simulink model "IRB140_speed"  (R2019a)
settings: Solver=VariableStepAuto  StartTime=0.0  StopTime=10.0  RelTol=1e-3
InitFcn:
  | rpm_max=5000;
  | trq_stall=7;
  | T_i=1e-3;
  | eta=100;
  | rpm_eta=3000;
  | trq_eta=2.07;
  | J=0.672*1e-4;
  | rpm0=0;
  | gearRatio=10;
  | ts=0.0025;
undefined symbols (not defined in the file or in its folder): sigbuilder_block, X, Y, Z
libraries: sm_lib x61, fl_lib x37, nesl_utility x31, simulink x12, eeGeneralControl x12, ee_lib x6
(part 1 of 3)
settings Model: Creator=Richard urben  LastModifiedBy=Richard urben

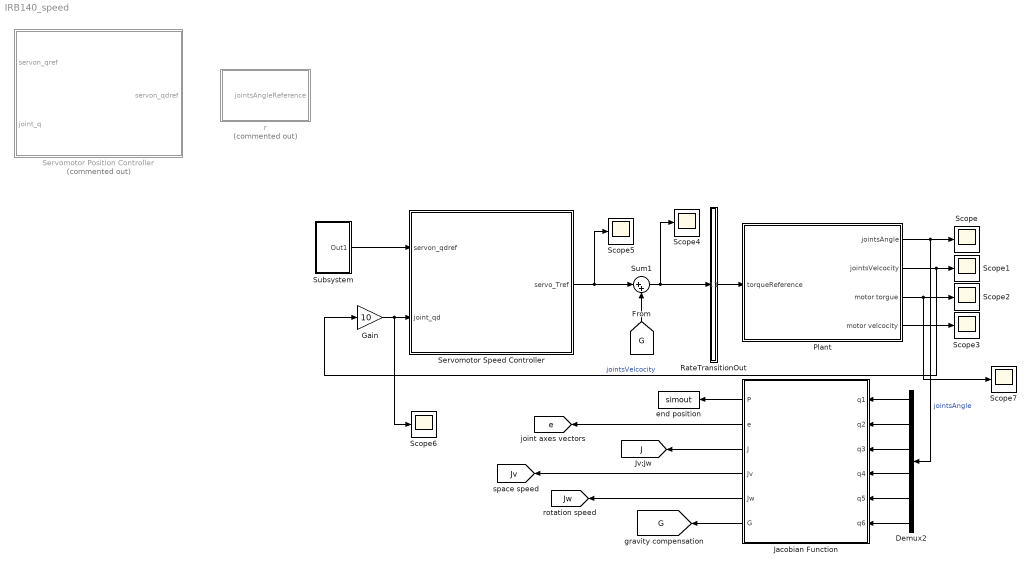
== system IRB140_speed ==
  Demux2 : Demux  Outputs=6
  Gain : Gain  Gain=10
  Jacobian Function : MATLAB Function  TreatAsAtomicUnit=on
  Plant : Subsystem
  RateTransitionOut : Subsystem
  Scope{,1..7} (8 alike) : Scope
  Servomotor Position Controller : Subsystem  Commented=on
  Servomotor Speed Controller : Subsystem
  Subsystem : Subsystem
  Sum1 : Sum  Inputs=|++
  "end position " : ToWorkspace  VariableName=simout  SaveFormat=Timeseries  SampleTime=-1
  r : Subsystem  Commented=on
      mask Display: disp('input')
  tag scope: G=global, J=global, Jv=global, Jw=global, e=global
  wires:
  Plant/2(jointsVelcocity) -> Gain/1, Scope1/1  "jointsVelcocity"
  RateTransitionOut/1(tRef) -> Plant/1(torqueReference)
  Plant/1(jointsAngle) -> Demux2/1, Scope/1  "jointsAngle"
  Plant/3(motor torgue) -> Scope7/1, Scope2/1
  Plant/4(motor velcocity) -> Scope3/1
  Demux2/5 -> Jacobian Function/5(q5)
  Demux2/3 -> Jacobian Function/3(q3)
  Demux2/2 -> Jacobian Function/2(q2)
  Demux2/4 -> Jacobian Function/4(q4)
  Demux2/1 -> Jacobian Function/1(q1)
  Demux2/6 -> Jacobian Function/6(q6)
  Jacobian Function/1(P) -> "end position "/1
  Jacobian Function/2(e) -> [e]
  Jacobian Function/3(J) -> [J]
  Jacobian Function/4(Jv) -> [Jv]
  Jacobian Function/5(Jw) -> [Jw]
  Jacobian Function/6(G) -> [G]
  Sum1/1 -> Scope4/1, RateTransitionOut/1(tRefIn)
  Servomotor Speed Controller/1(servo_Tref) -> Scope5/1, Sum1/1
  [G] -> Sum1/2
  Gain/1 -> Scope6/1, Servomotor Speed Controller/2(joint_qd)
  Subsystem/1(Out1) -> Servomotor Speed Controller/1(servon_qdref)

== system IRB140_speed/Plant ==
  torqueReference : Inport  Unit=N*m
  DC Voltage Source : fl_lib/Electrical/Electrical Sources/DC Voltage Source  v0=12 V
  ERef Vcc : fl_lib/Electrical/Electrical Elements/Electrical Reference
      settings: SourceProductName=Foundation Library
  MRRef Motor : fl_lib/Mechanical/Rotational Elements/Mechanical Rotational Reference
      settings: SourceProductName=Foundation Library
  robot : Subsystem
  servo system : Subsystem
  jointsAngle : Outport  Unit=deg
  jointsVelcocity : Outport  Port=2  Unit=deg/s
  motor torgue : Outport  Port=3
  motor velcocity : Outport  Port=4
  wires:
  robot/2(w) -> jointsVelcocity/1  "jointsvelocity"
  robot/1(q) -> jointsAngle/1  "jointsangle"
  servo system/1(torque) -> motor torgue/1  "motor torque"
  servo system/2(motVel) -> motor velcocity/1  "motor velocity"
  torqueReference/1 -> servo system/1(tRef)
  connections:
  robot/LConn4 -- servo system/RConn4
  robot/LConn5 -- servo system/RConn5
  robot/LConn3 -- servo system/RConn3
  robot/LConn1 -- servo system/RConn1
  robot/LConn6 -- servo system/RConn6
  servo system/RConn7 -- MRRef Motor/LConn1 -- robot/LConn7
  robot/LConn2 -- servo system/RConn2
  ERef Vcc/LConn1 -- DC Voltage Source/RConn1 -- servo system/LConn2
  DC Voltage Source/LConn1 -- servo system/LConn1

== system IRB140_speed/RateTransitionOut ==
  tRefIn : Inport  Unit=N*m
  Demux : Demux  Outputs=6
  Mux : Mux  Inputs=6
  Zero-Order Hold{,1..5} (6 alike) : ZeroOrderHold  SampleTime=-1
  tRef : Outport  SampleTime=0
  wires:
  Demux/3 -> Zero-Order Hold2/1
  tRefIn/1 -> Demux/1
  Demux/2 -> Zero-Order Hold1/1
  Demux/5 -> Zero-Order Hold4/1
  Demux/4 -> Zero-Order Hold3/1
  Demux/1 -> Zero-Order Hold/1
  Demux/6 -> Zero-Order Hold5/1
  Zero-Order Hold5/1 -> Mux/6
  Zero-Order Hold4/1 -> Mux/5
  Zero-Order Hold1/1 -> Mux/2
  Zero-Order Hold/1 -> Mux/1
  Zero-Order Hold2/1 -> Mux/3
  Zero-Order Hold3/1 -> Mux/4
  Mux/1 -> tRef/1

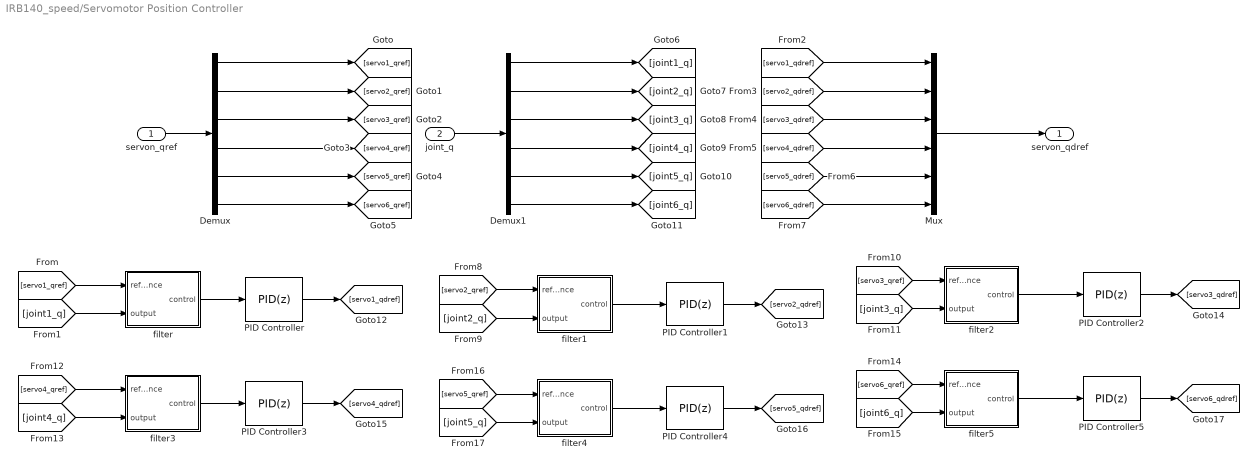
== system IRB140_speed/Servomotor Position Controller ==
  servon_qref : Inport  Unit=deg
  joint_q : Inport  Port=2  Unit=deg
  Demux : Demux  Outputs=6
  Demux1 : Demux  Outputs=6
  Mux : Mux  Inputs=6
  PID Controller : simulink/Continuous/PID Controller  Controller=PID  Form=Parallel  TimeDomain=Discrete-time  SampleTime=ts  IntegratorMethod=Forward Euler  FilterMethod=Forward Euler  ControllerParametersSource=internal  P=10.4951083286152  I=0.000420166597419455  D=-67.8994259865588  UseFilter=on  N=0.00133454786069086  TunerSelectOption=Transfer Function Based (PID Tuner App)  InitialConditionSource=internal  InitialConditionForIntegrator=0  InitialConditionForFilter=0  DifferentiatorICPrevScaledInput=0  ExternalReset=none  TrackingMode=off  Kt=1  LimitOutput=off  UpperSaturationLimit=inf  LowerSaturationLimit=-inf  LinearizeAsGain=on  AntiWindupMode=none  Kb=1  POutMin=[]  POutMax=[]  IOutMin=[]  IOutMax=[]  DOutMin=[]  DOutMax=[]  NOutMin=[]  NOutMax=[]  SumOutMin=[]  SumOutMax=[]  SaturationOutMin=[]  SaturationOutMax=[]  PParamMin=[]  PParamMax=[]  IParamMin=[]  IParamMax=[]  DParamMin=[]  DParamMax=[]  NParamMin=[]  NParamMax=[]  KbParamMin=[]  KbParamMax=[]  KtParamMin=[]  KtParamMax=[]  KbOutMin=[]  KbOutMax=[]  KtOutMin=[]  KtOutMax=[]  IntegratorOutMin=[]  IntegratorOutMax=[]  FilterOutMin=[]  FilterOutMax=[]  SumI1OutMin=[]  SumI1OutMax=[]  SumI2OutMin=[]  SumI2OutMax=[]  SumI3OutMin=[]  SumI3OutMax=[]  SumI4OutMin=[]  SumI4OutMax=[]  SumDOutMin=[]  SumDOutMax=[]  DifferentiatorOutMin=[]  DifferentiatorOutMax=[]  FilterDiffOutCoefMin=[]  FilterDiffOutCoefMax=[]  ReciprocalOutMin=[]  ReciprocalOutMax=[]  SumDenOutMin=[]  SumDenOutMax=[]  SumNumOutMin=[]  SumNumOutMax=[]  DivideOutMin=[]  DivideOutMax=[]  IntegratorContinuousStateAttributes=''  IntegratorStateMustResolveToSignalObject=off  IntegratorRTWStateStorageClass=Auto  FilterContinuousStateAttributes=''  FilterStateMustResolveToSignalObject=off  FilterRTWStateStorageClass=Auto  ParallelPVariant=InternalParameters  IdealPVariant=Disabled  IVariant=InternalParameters  DVariant=InternalParameters  IntegratorVariant=Discrete  SatVariant=Disabled  AWVariant=Passthrough  PCopyVariant=Disabled  TRVariant=Disabled  FdbkBlocksVariant=Forward  IdealPFdbkVariant=Disabled  SatFdbkVariant=Disabled  DerivativeFilterVariant=ForwardEulerFilter  NVariant=InternalParameters  NCopyVariant=Disabled  FilterICVariant=InternalICsFilter  IntegratorICVariant=InternalICs  ExternalResetVariant=Disabled  TRSumVariant=Passthrough  SumFdbkVariant=Disabled  SumVariant=Sum_PID
  PID Controller1 : simulink/Continuous/PID Controller  Controller=PID  Form=Parallel  TimeDomain=Discrete-time  SampleTime=ts  IntegratorMethod=Forward Euler  FilterMethod=Forward Euler  ControllerParametersSource=internal  P=3.54979973257463  I=0.000142016761735363  D=5.15669282783303  UseFilter=on  N=761.904761904762  TunerSelectOption=Transfer Function Based (PID Tuner App)  InitialConditionSource=internal  InitialConditionForIntegrator=0  InitialConditionForFilter=0  DifferentiatorICPrevScaledInput=0  ExternalReset=none  TrackingMode=off  Kt=1  LimitOutput=off  UpperSaturationLimit=inf  LowerSaturationLimit=-inf  LinearizeAsGain=on  AntiWindupMode=none  Kb=1  POutMin=[]  POutMax=[]  IOutMin=[]  IOutMax=[]  DOutMin=[]  DOutMax=[]  NOutMin=[]  NOutMax=[]  SumOutMin=[]  SumOutMax=[]  SaturationOutMin=[]  SaturationOutMax=[]  PParamMin=[]  PParamMax=[]  IParamMin=[]  IParamMax=[]  DParamMin=[]  DParamMax=[]  NParamMin=[]  NParamMax=[]  KbParamMin=[]  KbParamMax=[]  KtParamMin=[]  KtParamMax=[]  KbOutMin=[]  KbOutMax=[]  KtOutMin=[]  KtOutMax=[]  IntegratorOutMin=[]  IntegratorOutMax=[]  FilterOutMin=[]  FilterOutMax=[]  SumI1OutMin=[]  SumI1OutMax=[]  SumI2OutMin=[]  SumI2OutMax=[]  SumI3OutMin=[]  SumI3OutMax=[]  SumI4OutMin=[]  SumI4OutMax=[]  SumDOutMin=[]  SumDOutMax=[]  DifferentiatorOutMin=[]  DifferentiatorOutMax=[]  FilterDiffOutCoefMin=[]  FilterDiffOutCoefMax=[]  ReciprocalOutMin=[]  ReciprocalOutMax=[]  SumDenOutMin=[]  SumDenOutMax=[]  SumNumOutMin=[]  SumNumOutMax=[]  DivideOutMin=[]  DivideOutMax=[]  IntegratorContinuousStateAttributes=''  IntegratorStateMustResolveToSignalObject=off  IntegratorRTWStateStorageClass=Auto  FilterContinuousStateAttributes=''  FilterStateMustResolveToSignalObject=off  FilterRTWStateStorageClass=Auto  ParallelPVariant=InternalParameters  IdealPVariant=Disabled  IVariant=InternalParameters  DVariant=InternalParameters  IntegratorVariant=Discrete  SatVariant=Disabled  AWVariant=Passthrough  PCopyVariant=Disabled  TRVariant=Disabled  FdbkBlocksVariant=Forward  IdealPFdbkVariant=Disabled  SatFdbkVariant=Disabled  DerivativeFilterVariant=ForwardEulerFilter  NVariant=InternalParameters  NCopyVariant=Disabled  FilterICVariant=InternalICsFilter  IntegratorICVariant=InternalICs  ExternalResetVariant=Disabled  TRSumVariant=Passthrough  SumFdbkVariant=Disabled  SumVariant=Sum_PID
  PID Controller2 : simulink/Continuous/PID Controller  Controller=PID  Form=Parallel  TimeDomain=Discrete-time  SampleTime=ts  IntegratorMethod=Forward Euler  FilterMethod=Forward Euler  ControllerParametersSource=internal  P=-140.487680520088  I=93.0957479013491  D=581.760060440757  UseFilter=on  N=0.380969902119655  TunerSelectOption=Transfer Function Based (PID Tuner App)  InitialConditionSource=internal  InitialConditionForIntegrator=0  InitialConditionForFilter=0  DifferentiatorICPrevScaledInput=0  ExternalReset=none  TrackingMode=off  Kt=1  LimitOutput=off  UpperSaturationLimit=inf  LowerSaturationLimit=-inf  LinearizeAsGain=on  AntiWindupMode=none  Kb=1  POutMin=[]  POutMax=[]  IOutMin=[]  IOutMax=[]  DOutMin=[]  DOutMax=[]  NOutMin=[]  NOutMax=[]  SumOutMin=[]  SumOutMax=[]  SaturationOutMin=[]  SaturationOutMax=[]  PParamMin=[]  PParamMax=[]  IParamMin=[]  IParamMax=[]  DParamMin=[]  DParamMax=[]  NParamMin=[]  NParamMax=[]  KbParamMin=[]  KbParamMax=[]  KtParamMin=[]  KtParamMax=[]  KbOutMin=[]  KbOutMax=[]  KtOutMin=[]  KtOutMax=[]  IntegratorOutMin=[]  IntegratorOutMax=[]  FilterOutMin=[]  FilterOutMax=[]  SumI1OutMin=[]  SumI1OutMax=[]  SumI2OutMin=[]  SumI2OutMax=[]  SumI3OutMin=[]  SumI3OutMax=[]  SumI4OutMin=[]  SumI4OutMax=[]  SumDOutMin=[]  SumDOutMax=[]  DifferentiatorOutMin=[]  DifferentiatorOutMax=[]  FilterDiffOutCoefMin=[]  FilterDiffOutCoefMax=[]  ReciprocalOutMin=[]  ReciprocalOutMax=[]  SumDenOutMin=[]  SumDenOutMax=[]  SumNumOutMin=[]  SumNumOutMax=[]  DivideOutMin=[]  DivideOutMax=[]  IntegratorContinuousStateAttributes=''  IntegratorStateMustResolveToSignalObject=off  IntegratorRTWStateStorageClass=Auto  FilterContinuousStateAttributes=''  FilterStateMustResolveToSignalObject=off  FilterRTWStateStorageClass=Auto  ParallelPVariant=InternalParameters  IdealPVariant=Disabled  IVariant=InternalParameters  DVariant=InternalParameters  IntegratorVariant=Discrete  SatVariant=Disabled  AWVariant=Passthrough  PCopyVariant=Disabled  TRVariant=Disabled  FdbkBlocksVariant=Forward  IdealPFdbkVariant=Disabled  SatFdbkVariant=Disabled  DerivativeFilterVariant=ForwardEulerFilter  NVariant=InternalParameters  NCopyVariant=Disabled  FilterICVariant=InternalICsFilter  IntegratorICVariant=InternalICs  ExternalResetVariant=Disabled  TRSumVariant=Passthrough  SumFdbkVariant=Disabled  SumVariant=Sum_PID
  PID Controller3 : simulink/Continuous/PID Controller  Controller=PID  Form=Parallel  TimeDomain=Discrete-time  SampleTime=ts  IntegratorMethod=Forward Euler  FilterMethod=Forward Euler  ControllerParametersSource=internal  P=9.11824545476099  I=0.000364829647262142  D=0.827468756816228  UseFilter=on  N=735.731353896423  TunerSelectOption=Transfer Function Based (PID Tuner App)  InitialConditionSource=internal  InitialConditionForIntegrator=0  InitialConditionForFilter=0  DifferentiatorICPrevScaledInput=0  ExternalReset=none  TrackingMode=off  Kt=1  LimitOutput=off  UpperSaturationLimit=inf  LowerSaturationLimit=-inf  LinearizeAsGain=on  AntiWindupMode=none  Kb=1  POutMin=[]  POutMax=[]  IOutMin=[]  IOutMax=[]  DOutMin=[]  DOutMax=[]  NOutMin=[]  NOutMax=[]  SumOutMin=[]  SumOutMax=[]  SaturationOutMin=[]  SaturationOutMax=[]  PParamMin=[]  PParamMax=[]  IParamMin=[]  IParamMax=[]  DParamMin=[]  DParamMax=[]  NParamMin=[]  NParamMax=[]  KbParamMin=[]  KbParamMax=[]  KtParamMin=[]  KtParamMax=[]  KbOutMin=[]  KbOutMax=[]  KtOutMin=[]  KtOutMax=[]  IntegratorOutMin=[]  IntegratorOutMax=[]  FilterOutMin=[]  FilterOutMax=[]  SumI1OutMin=[]  SumI1OutMax=[]  SumI2OutMin=[]  SumI2OutMax=[]  SumI3OutMin=[]  SumI3OutMax=[]  SumI4OutMin=[]  SumI4OutMax=[]  SumDOutMin=[]  SumDOutMax=[]  DifferentiatorOutMin=[]  DifferentiatorOutMax=[]  FilterDiffOutCoefMin=[]  FilterDiffOutCoefMax=[]  ReciprocalOutMin=[]  ReciprocalOutMax=[]  SumDenOutMin=[]  SumDenOutMax=[]  SumNumOutMin=[]  SumNumOutMax=[]  DivideOutMin=[]  DivideOutMax=[]  IntegratorContinuousStateAttributes=''  IntegratorStateMustResolveToSignalObject=off  IntegratorRTWStateStorageClass=Auto  FilterContinuousStateAttributes=''  FilterStateMustResolveToSignalObject=off  FilterRTWStateStorageClass=Auto  ParallelPVariant=InternalParameters  IdealPVariant=Disabled  IVariant=InternalParameters  DVariant=InternalParameters  IntegratorVariant=Discrete  SatVariant=Disabled  AWVariant=Passthrough  PCopyVariant=Disabled  TRVariant=Disabled  FdbkBlocksVariant=Forward  IdealPFdbkVariant=Disabled  SatFdbkVariant=Disabled  DerivativeFilterVariant=ForwardEulerFilter  NVariant=InternalParameters  NCopyVariant=Disabled  FilterICVariant=InternalICsFilter  IntegratorICVariant=InternalICs  ExternalResetVariant=Disabled  TRSumVariant=Passthrough  SumFdbkVariant=Disabled  SumVariant=Sum_PID
  PID Controller4 : simulink/Continuous/PID Controller  Controller=PID  Form=Parallel  TimeDomain=Discrete-time  SampleTime=ts  IntegratorMethod=Forward Euler  FilterMethod=Forward Euler  ControllerParametersSource=internal  P=9.17149127904828  I=0.0429049056469866  D=39.4802374585805  UseFilter=on  N=0.0426490330143886  TunerSelectOption=Transfer Function Based (PID Tuner App)  InitialConditionSource=internal  InitialConditionForIntegrator=0  InitialConditionForFilter=0  DifferentiatorICPrevScaledInput=0  ExternalReset=none  TrackingMode=off  Kt=1  LimitOutput=off  UpperSaturationLimit=inf  LowerSaturationLimit=-inf  LinearizeAsGain=on  AntiWindupMode=none  Kb=1  POutMin=[]  POutMax=[]  IOutMin=[]  IOutMax=[]  DOutMin=[]  DOutMax=[]  NOutMin=[]  NOutMax=[]  SumOutMin=[]  SumOutMax=[]  SaturationOutMin=[]  SaturationOutMax=[]  PParamMin=[]  PParamMax=[]  IParamMin=[]  IParamMax=[]  DParamMin=[]  DParamMax=[]  NParamMin=[]  NParamMax=[]  KbParamMin=[]  KbParamMax=[]  KtParamMin=[]  KtParamMax=[]  KbOutMin=[]  KbOutMax=[]  KtOutMin=[]  KtOutMax=[]  IntegratorOutMin=[]  IntegratorOutMax=[]  FilterOutMin=[]  FilterOutMax=[]  SumI1OutMin=[]  SumI1OutMax=[]  SumI2OutMin=[]  SumI2OutMax=[]  SumI3OutMin=[]  SumI3OutMax=[]  SumI4OutMin=[]  SumI4OutMax=[]  SumDOutMin=[]  SumDOutMax=[]  DifferentiatorOutMin=[]  DifferentiatorOutMax=[]  FilterDiffOutCoefMin=[]  FilterDiffOutCoefMax=[]  ReciprocalOutMin=[]  ReciprocalOutMax=[]  SumDenOutMin=[]  SumDenOutMax=[]  SumNumOutMin=[]  SumNumOutMax=[]  DivideOutMin=[]  DivideOutMax=[]  IntegratorContinuousStateAttributes=''  IntegratorStateMustResolveToSignalObject=off  IntegratorRTWStateStorageClass=Auto  FilterContinuousStateAttributes=''  FilterStateMustResolveToSignalObject=off  FilterRTWStateStorageClass=Auto  ParallelPVariant=InternalParameters  IdealPVariant=Disabled  IVariant=InternalParameters  DVariant=InternalParameters  IntegratorVariant=Discrete  SatVariant=Disabled  AWVariant=Passthrough  PCopyVariant=Disabled  TRVariant=Disabled  FdbkBlocksVariant=Forward  IdealPFdbkVariant=Disabled  SatFdbkVariant=Disabled  DerivativeFilterVariant=ForwardEulerFilter  NVariant=InternalParameters  NCopyVariant=Disabled  FilterICVariant=InternalICsFilter  IntegratorICVariant=InternalICs  ExternalResetVariant=Disabled  TRSumVariant=Passthrough  SumFdbkVariant=Disabled  SumVariant=Sum_PID
  PID Controller5 : simulink/Continuous/PID Controller  Controller=PID  Form=Parallel  TimeDomain=Discrete-time  SampleTime=ts  IntegratorMethod=Forward Euler  FilterMethod=Forward Euler  ControllerParametersSource=internal  P=10.2886368566018  I=0.000521762347061113  D=0.264911949905084  UseFilter=on  N=7.86122759975994  TunerSelectOption=Transfer Function Based (PID Tuner App)  InitialConditionSource=internal  InitialConditionForIntegrator=0  InitialConditionForFilter=0  DifferentiatorICPrevScaledInput=0  ExternalReset=none  TrackingMode=off  Kt=1  LimitOutput=off  UpperSaturationLimit=inf  LowerSaturationLimit=-inf  LinearizeAsGain=on  AntiWindupMode=none  Kb=1  POutMin=[]  POutMax=[]  IOutMin=[]  IOutMax=[]  DOutMin=[]  DOutMax=[]  NOutMin=[]  NOutMax=[]  SumOutMin=[]  SumOutMax=[]  SaturationOutMin=[]  SaturationOutMax=[]  PParamMin=[]  PParamMax=[]  IParamMin=[]  IParamMax=[]  DParamMin=[]  DParamMax=[]  NParamMin=[]  NParamMax=[]  KbParamMin=[]  KbParamMax=[]  KtParamMin=[]  KtParamMax=[]  KbOutMin=[]  KbOutMax=[]  KtOutMin=[]  KtOutMax=[]  IntegratorOutMin=[]  IntegratorOutMax=[]  FilterOutMin=[]  FilterOutMax=[]  SumI1OutMin=[]  SumI1OutMax=[]  SumI2OutMin=[]  SumI2OutMax=[]  SumI3OutMin=[]  SumI3OutMax=[]  SumI4OutMin=[]  SumI4OutMax=[]  SumDOutMin=[]  SumDOutMax=[]  DifferentiatorOutMin=[]  DifferentiatorOutMax=[]  FilterDiffOutCoefMin=[]  FilterDiffOutCoefMax=[]  ReciprocalOutMin=[]  ReciprocalOutMax=[]  SumDenOutMin=[]  SumDenOutMax=[]  SumNumOutMin=[]  SumNumOutMax=[]  DivideOutMin=[]  DivideOutMax=[]  IntegratorContinuousStateAttributes=''  IntegratorStateMustResolveToSignalObject=off  IntegratorRTWStateStorageClass=Auto  FilterContinuousStateAttributes=''  FilterStateMustResolveToSignalObject=off  FilterRTWStateStorageClass=Auto  ParallelPVariant=InternalParameters  IdealPVariant=Disabled  IVariant=InternalParameters  DVariant=InternalParameters  IntegratorVariant=Discrete  SatVariant=Disabled  AWVariant=Passthrough  PCopyVariant=Disabled  TRVariant=Disabled  FdbkBlocksVariant=Forward  IdealPFdbkVariant=Disabled  SatFdbkVariant=Disabled  DerivativeFilterVariant=ForwardEulerFilter  NVariant=InternalParameters  NCopyVariant=Disabled  FilterICVariant=InternalICsFilter  IntegratorICVariant=InternalICs  ExternalResetVariant=Disabled  TRSumVariant=Passthrough  SumFdbkVariant=Disabled  SumVariant=Sum_PID
  filter : Subsystem
  filter1 : Subsystem
  filter2 : Subsystem
  filter3 : Subsystem
  filter4 : Subsystem
  filter5 : Subsystem
  servon_qdref : Outport  Unit=deg/s
  wires:
  PID Controller/1 -> [servo1_qdref]
  [joint5_q] -> filter4/2(output)
  Demux/3 -> [servo3_qref]
  Demux/6 -> [servo6_qref]
  Demux/5 -> [servo5_qref]
  Demux/4 -> [servo4_qref]
  Demux1/3 -> [joint3_q]
  Demux/2 -> [servo2_qref]
  filter4/1(control) -> PID Controller4/1
  [servo2_qdref] -> Mux/2
  Demux1/2 -> [joint2_q]
  joint_q/1 -> Demux1/1
  Demux/1 -> [servo1_qref]
  [servo1_qref] -> filter/1(reference)
  Demux1/6 -> [joint6_q]
  [servo2_qref] -> filter1/1(reference)
  filter3/1(control) -> PID Controller3/1
  [joint6_q] -> filter5/2(output)
  Demux1/4 -> [joint4_q]
  servon_qref/1 -> Demux/1
  Demux1/5 -> [joint5_q]
  filter/1(control) -> PID Controller/1
  Demux1/1 -> [joint1_q]
  PID Controller5/1 -> [servo6_qdref]
  [servo1_qdref] -> Mux/1
  PID Controller2/1 -> [servo3_qdref]
  [servo5_qdref] -> Mux/5
  [servo4_qdref] -> Mux/4
  [servo6_qdref] -> Mux/6
  [servo3_qdref] -> Mux/3
  [joint1_q] -> filter/2(output)
  [joint2_q] -> filter1/2(output)
  Mux/1 -> servon_qdref/1
  PID Controller1/1 -> [servo2_qdref]
  filter1/1(control) -> PID Controller1/1
  filter2/1(control) -> PID Controller2/1
  PID Controller3/1 -> [servo4_qdref]
  PID Controller4/1 -> [servo5_qdref]
  [servo6_qref] -> filter5/1(reference)
  [servo5_qref] -> filter4/1(reference)
  [joint3_q] -> filter2/2(output)
  [servo3_qref] -> filter2/1(reference)
  [servo4_qref] -> filter3/1(reference)
  [joint4_q] -> filter3/2(output)
  filter5/1(control) -> PID Controller5/1

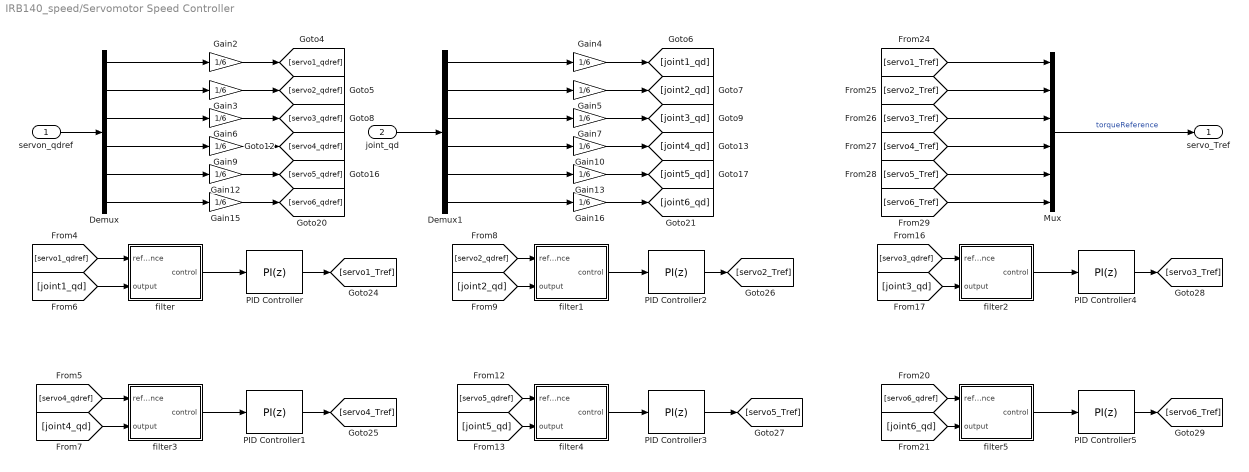
== system IRB140_speed/Servomotor Speed Controller ==
  servon_qdref : Inport
  joint_qd : Inport  Port=2
  Demux : Demux  Outputs=6
  Demux1 : Demux  Outputs=6
  Gain{2..7,9..10,12..13,15..16} (12 alike) : Gain  Gain=1/6
  Mux : Mux  Inputs=6
  PID Controller{,1..3} (4 alike) : simulink/Continuous/PID Controller  Controller=PI  Form=Parallel  TimeDomain=Discrete-time  SampleTime=ts  IntegratorMethod=Forward Euler  FilterMethod=Forward Euler  ControllerParametersSource=internal  P=5  I=0  D=0  UseFilter=on  N=0  TunerSelectOption=Transfer Function Based (PID Tuner App)  InitialConditionSource=internal  InitialConditionForIntegrator=0  InitialConditionForFilter=0  DifferentiatorICPrevScaledInput=0  ExternalReset=none  TrackingMode=off  Kt=1  LimitOutput=off  UpperSaturationLimit=inf  LowerSaturationLimit=-inf  LinearizeAsGain=on  AntiWindupMode=none  Kb=1  POutMin=[]  POutMax=[]  IOutMin=[]  IOutMax=[]  DOutMin=[]  DOutMax=[]  NOutMin=[]  NOutMax=[]  SumOutMin=[]  SumOutMax=[]  SaturationOutMin=[]  SaturationOutMax=[]  PParamMin=[]  PParamMax=[]  IParamMin=[]  IParamMax=[]  DParamMin=[]  DParamMax=[]  NParamMin=[]  NParamMax=[]  KbParamMin=[]  KbParamMax=[]  KtParamMin=[]  KtParamMax=[]  KbOutMin=[]  KbOutMax=[]  KtOutMin=[]  KtOutMax=[]  IntegratorOutMin=[]  IntegratorOutMax=[]  FilterOutMin=[]  FilterOutMax=[]  SumI1OutMin=[]  SumI1OutMax=[]  SumI2OutMin=[]  SumI2OutMax=[]  SumI3OutMin=[]  SumI3OutMax=[]  SumI4OutMin=[]  SumI4OutMax=[]  SumDOutMin=[]  SumDOutMax=[]  DifferentiatorOutMin=[]  DifferentiatorOutMax=[]  FilterDiffOutCoefMin=[]  FilterDiffOutCoefMax=[]  ReciprocalOutMin=[]  ReciprocalOutMax=[]  SumDenOutMin=[]  SumDenOutMax=[]  SumNumOutMin=[]  SumNumOutMax=[]  DivideOutMin=[]  DivideOutMax=[]  IntegratorContinuousStateAttributes=''  IntegratorStateMustResolveToSignalObject=off  IntegratorRTWStateStorageClass=Auto  FilterContinuousStateAttributes=''  FilterStateMustResolveToSignalObject=off  FilterRTWStateStorageClass=Auto  ParallelPVariant=InternalParameters  IdealPVariant=Disabled  IVariant=InternalParameters  DVariant=Disabled  IntegratorVariant=Discrete  SatVariant=Disabled  AWVariant=Passthrough  PCopyVariant=Disabled  TRVariant=Disabled  FdbkBlocksVariant=Forward  IdealPFdbkVariant=Disabled  SatFdbkVariant=Disabled  DerivativeFilterVariant=Disabled  NVariant=Disabled  NCopyVariant=Disabled_SignalSpec  FilterICVariant=Disabled  IntegratorICVariant=InternalICs  ExternalResetVariant=Disabled  TRSumVariant=Passthrough  SumFdbkVariant=Disabled  SumVariant=Sum_PI
  PID Controller4 : simulink/Continuous/PID Controller  Controller=PI  Form=Parallel  TimeDomain=Discrete-time  SampleTime=ts  IntegratorMethod=Forward Euler  FilterMethod=Forward Euler  ControllerParametersSource=internal  P=5  I=0  D=0  UseFilter=on  N=0  TunerSelectOption=Transfer Function Based (PID Tuner App)  InitialConditionSource=internal  InitialConditionForIntegrator=0  InitialConditionForFilter=0  DifferentiatorICPrevScaledInput=0  ExternalReset=none  TrackingMode=off  Kt=1  LimitOutput=off  UpperSaturationLimit=0.001  LowerSaturationLimit=-0.001  LinearizeAsGain=on  AntiWindupMode=none  Kb=1  POutMin=[]  POutMax=[]  IOutMin=[]  IOutMax=[]  DOutMin=[]  DOutMax=[]  NOutMin=[]  NOutMax=[]  SumOutMin=[]  SumOutMax=[]  SaturationOutMin=[]  SaturationOutMax=[]  PParamMin=[]  PParamMax=[]  IParamMin=[]  IParamMax=[]  DParamMin=[]  DParamMax=[]  NParamMin=[]  NParamMax=[]  KbParamMin=[]  KbParamMax=[]  KtParamMin=[]  KtParamMax=[]  KbOutMin=[]  KbOutMax=[]  KtOutMin=[]  KtOutMax=[]  IntegratorOutMin=[]  IntegratorOutMax=[]  FilterOutMin=[]  FilterOutMax=[]  SumI1OutMin=[]  SumI1OutMax=[]  SumI2OutMin=[]  SumI2OutMax=[]  SumI3OutMin=[]  SumI3OutMax=[]  SumI4OutMin=[]  SumI4OutMax=[]  SumDOutMin=[]  SumDOutMax=[]  DifferentiatorOutMin=[]  DifferentiatorOutMax=[]  FilterDiffOutCoefMin=[]  FilterDiffOutCoefMax=[]  ReciprocalOutMin=[]  ReciprocalOutMax=[]  SumDenOutMin=[]  SumDenOutMax=[]  SumNumOutMin=[]  SumNumOutMax=[]  DivideOutMin=[]  DivideOutMax=[]  IntegratorContinuousStateAttributes=''  IntegratorStateMustResolveToSignalObject=off  IntegratorRTWStateStorageClass=Auto  FilterContinuousStateAttributes=''  FilterStateMustResolveToSignalObject=off  FilterRTWStateStorageClass=Auto  ParallelPVariant=InternalParameters  IdealPVariant=Disabled  IVariant=InternalParameters  DVariant=Disabled  IntegratorVariant=Discrete  SatVariant=Disabled  AWVariant=Passthrough  PCopyVariant=Disabled  TRVariant=Disabled  FdbkBlocksVariant=Forward  IdealPFdbkVariant=Disabled  SatFdbkVariant=Disabled  DerivativeFilterVariant=Disabled  NVariant=Disabled  NCopyVariant=Disabled_SignalSpec  FilterICVariant=Disabled  IntegratorICVariant=InternalICs  ExternalResetVariant=Disabled  TRSumVariant=Passthrough  SumFdbkVariant=Disabled  SumVariant=Sum_PI
  PID Controller5 : simulink/Continuous/PID Controller  Controller=PI  Form=Parallel  TimeDomain=Discrete-time  SampleTime=ts  IntegratorMethod=Forward Euler  FilterMethod=Forward Euler  ControllerParametersSource=internal  P=5  I=0  D=0  UseFilter=on  N=0  TunerSelectOption=Transfer Function Based (PID Tuner App)  InitialConditionSource=internal  InitialConditionForIntegrator=0  InitialConditionForFilter=0  DifferentiatorICPrevScaledInput=0  ExternalReset=none  TrackingMode=off  Kt=1  LimitOutput=off  UpperSaturationLimit=0.001  LowerSaturationLimit=-0.001  LinearizeAsGain=on  AntiWindupMode=none  Kb=1  POutMin=[]  POutMax=[]  IOutMin=[]  IOutMax=[]  DOutMin=[]  DOutMax=[]  NOutMin=[]  NOutMax=[]  SumOutMin=[]  SumOutMax=[]  SaturationOutMin=[]  SaturationOutMax=[]  PParamMin=[]  PParamMax=[]  IParamMin=[]  IParamMax=[]  DParamMin=[]  DParamMax=[]  NParamMin=[]  NParamMax=[]  KbParamMin=[]  KbParamMax=[]  KtParamMin=[]  KtParamMax=[]  KbOutMin=[]  KbOutMax=[]  KtOutMin=[]  KtOutMax=[]  IntegratorOutMin=[]  IntegratorOutMax=[]  FilterOutMin=[]  FilterOutMax=[]  SumI1OutMin=[]  SumI1OutMax=[]  SumI2OutMin=[]  SumI2OutMax=[]  SumI3OutMin=[]  SumI3OutMax=[]  SumI4OutMin=[]  SumI4OutMax=[]  SumDOutMin=[]  SumDOutMax=[]  DifferentiatorOutMin=[]  DifferentiatorOutMax=[]  FilterDiffOutCoefMin=[]  FilterDiffOutCoefMax=[]  ReciprocalOutMin=[]  ReciprocalOutMax=[]  SumDenOutMin=[]  SumDenOutMax=[]  SumNumOutMin=[]  SumNumOutMax=[]  DivideOutMin=[]  DivideOutMax=[]  IntegratorContinuousStateAttributes=''  IntegratorStateMustResolveToSignalObject=off  IntegratorRTWStateStorageClass=Auto  FilterContinuousStateAttributes=''  FilterStateMustResolveToSignalObject=off  FilterRTWStateStorageClass=Auto  ParallelPVariant=InternalParameters  IdealPVariant=Disabled  IVariant=InternalParameters  DVariant=Disabled  IntegratorVariant=Discrete  SatVariant=Disabled  AWVariant=Passthrough  PCopyVariant=Disabled  TRVariant=Disabled  FdbkBlocksVariant=Forward  IdealPFdbkVariant=Disabled  SatFdbkVariant=Disabled  DerivativeFilterVariant=Disabled  NVariant=Disabled  NCopyVariant=Disabled_SignalSpec  FilterICVariant=Disabled  IntegratorICVariant=InternalICs  ExternalResetVariant=Disabled  TRSumVariant=Passthrough  SumFdbkVariant=Disabled  SumVariant=Sum_PI
  filter : Subsystem
  filter1 : Subsystem
  filter2 : Subsystem
  filter3 : Subsystem
  filter4 : Subsystem
  filter5 : Subsystem
  servo_Tref : Outport  Unit=N*m
  wires:
  [servo1_qdref] -> filter/1(reference)
  [servo1_Tref] -> Mux/1
  Demux1/1 -> Gain4/1
  Gain2/1 -> [servo1_qdref]
  Gain6/1 -> [servo3_qdref]
  Gain12/1 -> [servo5_qdref]
  filter4/1(control) -> PID Controller3/1
  Gain15/1 -> [servo6_qdref]
  Demux/5 -> Gain12/1
  Gain5/1 -> [joint2_qd]
  Demux1/4 -> Gain10/1
  Gain13/1 -> [joint5_qd]
  Gain16/1 -> [joint6_qd]
  PID Controller5/1 -> [servo6_Tref]
  [servo6_qdref] -> filter5/1(reference)
  Gain10/1 -> [joint4_qd]
  [servo2_qdref] -> filter1/1(reference)
  Demux1/6 -> Gain16/1
  [servo2_Tref] -> Mux/2
  Gain3/1 -> [servo2_qdref]
  Gain9/1 -> [servo4_qdref]
  Gain7/1 -> [joint3_qd]
  [joint3_qd] -> filter2/2(output)
  Gain4/1 -> [joint1_qd]
  filter1/1(control) -> PID Controller2/1
  [servo4_Tref] -> Mux/4
  [joint5_qd] -> filter4/2(output)
  [servo3_Tref] -> Mux/3
  Demux1/5 -> Gain13/1
  Demux1/2 -> Gain5/1
  Demux/4 -> Gain9/1
  Mux/1 -> servo_Tref/1  "torqueReference"
  joint_qd/1 -> Demux1/1
  [servo4_qdref] -> filter3/1(reference)
  Demux1/3 -> Gain7/1
  [servo3_qdref] -> filter2/1(reference)
  [servo5_Tref] -> Mux/5
  [servo6_Tref] -> Mux/6
  servon_qdref/1 -> Demux/1
  Demux/1 -> Gain2/1
  Demux/6 -> Gain15/1
  [joint2_qd] -> filter1/2(output)
  [joint6_qd] -> filter5/2(output)
  Demux/2 -> Gain3/1
  Demux/3 -> Gain6/1
  PID Controller3/1 -> [servo5_Tref]
  PID Controller2/1 -> [servo2_Tref]
  filter5/1(control) -> PID Controller5/1
  PID Controller4/1 -> [servo3_Tref]
  filter2/1(control) -> PID Controller4/1
  PID Controller1/1 -> [servo4_Tref]
  filter3/1(control) -> PID Controller1/1
  PID Controller/1 -> [servo1_Tref]
  filter/1(control) -> PID Controller/1
  [joint4_qd] -> filter3/2(output)
  [joint1_qd] -> filter/2(output)
  [servo5_qdref] -> filter4/1(reference)

== system IRB140_speed/Subsystem ==
  Constant : Constant  Value=2000
  Constant{1..4,6} (5 alike) : Constant  Value=0
  Mux : Mux  Inputs=6
  Out1 : Outport
  wires:
  Mux/1 -> Out1/1
  Constant/1 -> Mux/1
  Constant2/1 -> Mux/2
  Constant1/1 -> Mux/3
  Constant3/1 -> Mux/4
  Constant6/1 -> Mux/5
  Constant4/1 -> Mux/6

== system IRB140_speed/r ==
  Mux : Mux  Inputs=6
  Mux1 : Mux  Commented=on  Inputs=6
  Subsystem : Subsystem  Commented=on
  Trajectories1 : Subsystem  Tag=STV Subsys  LoadFcn=sigbuilder_block('load');  StartFcn=sigbuilder_block('start');  StopFcn=sigbuilder_block('stop');  ClipboardFcn=sigbuilder_block('clipboard');  mask(Sigbuilder block){tuvar=[0:10]}
      mask help: Simulink:masks:SigbuilderBlock_MD
      mask init:
      | if ~strcmp(get_param(bdroot(gcbh),'SimulationStatus'),'stopped') tuvar = sigbuilder_block('maskInit'); end
      settings: CopyFcn=sigbuilder_block('copy');  DeleteFcn=sigbuilder_block('delete');  ModelCloseFcn=sigbuilder_block('modelClose');  PreSaveFcn=sigbuilder_block('preSave');  PauseFcn=sigbuilder_block('pause');  ContinueFcn=sigbuilder_block('continue');  NameChangeFcn=sigbuilder_block('namechange');  OpenFcn=sigbuilder_block('open',[6 30 1248 681 ]);  CloseFcn=sigbuilder_block('close');
      mask Display: plot(0, 0, 100, 100,[2, 2, 32, 32, 2], [68, 8, 8, 68, 68],[32, 2], [38, 38], [32, 19, 2],[53, 60, 44], [32, 17, 17, 2],[16, 16, 31, 31]);txt = getActiveGroup(gcbh);text(2, 100, txt,'verticalAlignment', 'top');
  jointsAngleReference : Outport
  wires:
  Trajectories1/6(servopos6) -> Mux/6
  Trajectories1/2(servopos2) -> Mux/2
  Trajectories1/5(servopos5) -> Mux/5
  Trajectories1/1(servopos1) -> Mux/1
  Trajectories1/4(servopos4) -> Mux/4
  Trajectories1/3(servopos3) -> Mux/3
  Subsystem/5(Out5) -> Mux1/5
  Subsystem/1(Out1) -> Mux1/1
  Subsystem/3(Out3) -> Mux1/3
  Subsystem/2(Out2) -> Mux1/2
  Subsystem/6(Out6) -> Mux1/6
  Subsystem/4(Out4) -> Mux1/4
  Mux/1 -> jointsAngleReference/1  "jointsAngleReference"

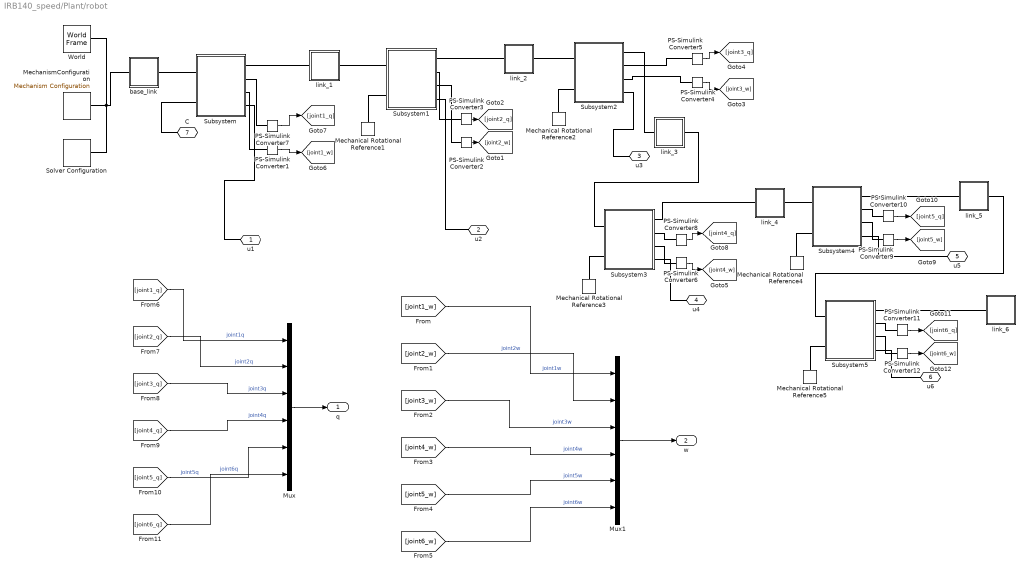
== system IRB140_speed/Plant/robot ==
  Mechanical Rotational Reference{1..5} (5 alike) : fl_lib/Mechanical/Rotational Elements/Mechanical Rotational Reference
  MechanismConfiguration : sm_lib/Utilities/Mechanism Configuration  UniformGravity=Constant  GravityVector=[0 0 -9.80665]  GravityUnits=m/s^2  LinearizationDelta=0.001
  Mux : Mux  Inputs=6
  Mux1 : Mux  Inputs=6
  PS-Simulink Converter{1..2,4,6,9,12} (6 alike) : nesl_utility/PS-Simulink Converter  PhysicalDomain=network_engine_domain  SubClassName=ps_output  LeftPortType=input  RightPortType=output  PseudoPeriodic=off  Frequencies=[]  Unit=deg/s  AffineConversion=off
  PS-Simulink Converter{3,5,7..8,10..11} (6 alike) : nesl_utility/PS-Simulink Converter  PhysicalDomain=network_engine_domain  SubClassName=ps_output  LeftPortType=input  RightPortType=output  PseudoPeriodic=off  Frequencies=[]  Unit=deg  AffineConversion=off
  Solver Configuration : nesl_utility/Solver Configuration  PhysicalDomain=network_engine_domain  SubClassName=solver  LeftPortType=input  RightPortType=generic  Tones=[]  Harmonics=[]  SimulateNoise=off  Profile=off  UseLocalSampling=off  EnableSwitchedLinearOptims=on  FrequencyDomain=off  UseCCode=off  RelTol=0.001  AbsTol=1e-06  MinStep=1e-09  ToWorkspace=off  RevertToSquareIcSolve=off  NumHomotopyIterations=100  PhasorMode=off  PhasorModeNumHarmonics=1  DoDC=off  ResidualTolerance=1e-09  UseLocalSolver=off  LocalSolverChoice=NE_BACKWARD_EULER_ADVANCER  LocalSolverSampleTime=0.001  DoFixedCost=off  MaxNonlinIter=3  MaxModeIter=2  LinearAlgebra=auto  EquationFormulation=NE_TIME_EF  DelaysMemoryBudget=1024  AutomaticFiltering=on  FilteringTimeConstant=0.001  PartitionStorageMethod=AS_NEEDED  PartitionMemoryBudget=1024  PartitionMethod=ROBUST
  Subsystem : Subsystem
  Subsystem1 : Subsystem
  Subsystem2 : Subsystem
  Subsystem3 : Subsystem
  Subsystem4 : Subsystem
  Subsystem5 : Subsystem
  World : sm_lib/Frames and Transforms/World Frame
  base_link : Subsystem
  link_1 : Subsystem
  link_2 : Subsystem
  link_3 : Subsystem
  link_4 : Subsystem
  link_5 : Subsystem
  link_6 : Subsystem
  u1 : PMIOPort  Side=Left
  u2 : PMIOPort  Port=2  Side=Left
  u3 : PMIOPort  Port=3  Side=Left
  u4 : PMIOPort  Port=4  Side=Left
  u5 : PMIOPort  Port=5  Side=Left
  u6 : PMIOPort  Port=6  Side=Left
  C : PMIOPort  Port=7  Side=Left
  q : Outport  Unit=deg
  w : Outport  Port=2  Unit=deg/s
  wires:
  [joint2_w] -> Mux1/2  "joint2w"
  PS-Simulink Converter1/1 -> [joint1_w]
  [joint4_q] -> Mux/4  "joint4q"
  [joint6_w] -> Mux1/6  "joint6w"
  PS-Simulink Converter8/1 -> [joint4_q]
  PS-Simulink Converter4/1 -> [joint3_w]
  [joint1_w] -> Mux1/1  "joint1w"
  [joint2_q] -> Mux/2  "joint2q"
  PS-Simulink Converter12/1 -> [joint6_w]
  PS-Simulink Converter11/1 -> [joint6_q]
  [joint5_q] -> Mux/5  "joint5q"
  [joint6_q] -> Mux/6  "joint6q"
  Mux1/1 -> w/1
  PS-Simulink Converter3/1 -> [joint2_q]
  [joint1_q] -> Mux/1  "joint1q"
  [joint3_q] -> Mux/3  "joint3q"
  PS-Simulink Converter9/1 -> [joint5_w]
  PS-Simulink Converter7/1 -> [joint1_q]
  PS-Simulink Converter10/1 -> [joint5_q]
  [joint5_w] -> Mux1/5  "joint5w"
  PS-Simulink Converter5/1 -> [joint3_q]
  Mux/1 -> q/1
  PS-Simulink Converter6/1 -> [joint4_w]
  PS-Simulink Converter2/1 -> [joint2_w]
  [joint4_w] -> Mux1/4  "joint4w"
  [joint3_w] -> Mux1/3  "joint3w"
  connections:
  Subsystem4/LConn1 -- link_4/RConn1
  World/RConn1 -- MechanismConfiguration/RConn1 -- Solver Configuration/RConn1 -- base_link/LConn1
  Mechanical Rotational Reference3/LConn1 -- Subsystem3/LConn2
  Subsystem4/RConn1 -- link_5/LConn1
  PS-Simulink Converter8/LConn1 -- Subsystem3/RConn2
  u4/RConn1 -- Subsystem3/RConn4
  PS-Simulink Converter12/LConn1 -- Subsystem5/RConn3
  PS-Simulink Converter11/LConn1 -- Subsystem5/RConn2
  Mechanical Rotational Reference4/LConn1 -- Subsystem4/LConn2
  PS-Simulink Converter1/LConn1 -- Subsystem/RConn3
  Mechanical Rotational Reference5/LConn1 -- Subsystem5/LConn2
  u3/RConn1 -- Subsystem2/RConn4
  Subsystem2/LConn1 -- link_2/RConn1
  u2/RConn1 -- Subsystem1/RConn4
  C/RConn1 -- Subsystem/LConn2
  Subsystem2/RConn1 -- link_3/LConn1
  PS-Simulink Converter10/LConn1 -- Subsystem4/RConn2
  PS-Simulink Converter6/LConn1 -- Subsystem3/RConn3
  u5/RConn1 -- Subsystem4/RConn4
  PS-Simulink Converter3/LConn1 -- Subsystem1/RConn2
  PS-Simulink Converter7/LConn1 -- Subsystem/RConn2
  PS-Simulink Converter5/LConn1 -- Subsystem2/RConn2
  link_2/LConn1 -- Subsystem1/RConn1
  Subsystem3/RConn1 -- link_4/LConn1
  link_1/RConn1 -- Subsystem1/LConn1
  base_link/RConn1 -- Subsystem/LConn1
  PS-Simulink Converter2/LConn1 -- Subsystem1/RConn3
  Subsystem3/LConn1 -- link_3/RConn1
  Subsystem/RConn1 -- link_1/LConn1
  Subsystem5/LConn1 -- link_5/RConn1
  PS-Simulink Converter9/LConn1 -- Subsystem4/RConn3
  u1/RConn1 -- Subsystem/RConn4
  PS-Simulink Converter4/LConn1 -- Subsystem2/RConn3
  u6/RConn1 -- Subsystem5/RConn4
  Subsystem5/RConn1 -- link_6/LConn1
  Mechanical Rotational Reference2/LConn1 -- Subsystem2/LConn2
  Subsystem1/LConn2 -- Mechanical Rotational Reference1/LConn1

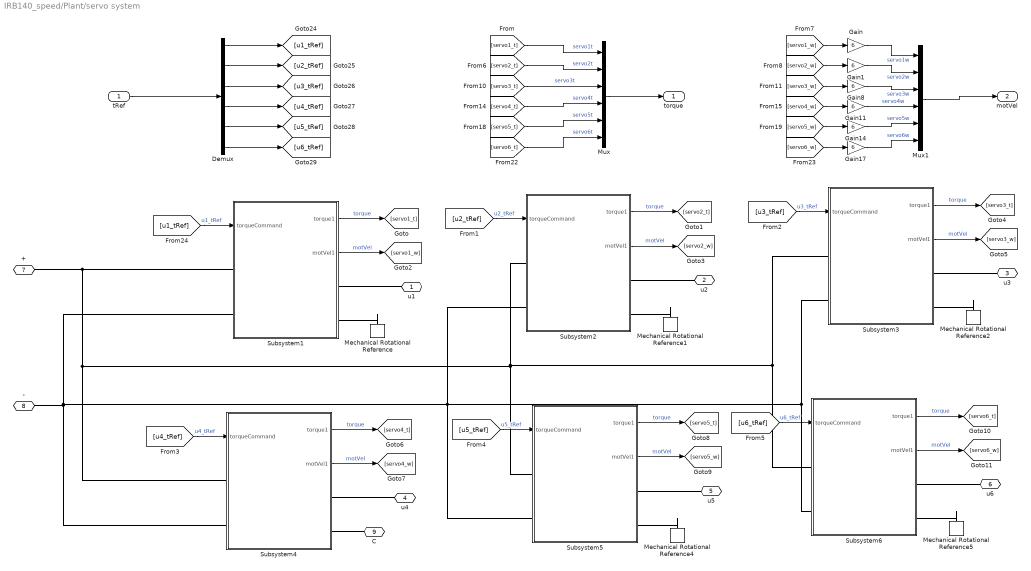
== system IRB140_speed/Plant/servo system ==
  tRef : Inport  Unit=N*m
  Demux : Demux  Outputs=6
  Gain{,1,8,11,14,17} (6 alike) : Gain  Gain=6
  Mechanical Rotational Reference{,1..2,4..5} (5 alike) : fl_lib/Mechanical/Rotational Elements/Mechanical Rotational Reference
  Mux : Mux  Inputs=6
  Mux1 : Mux  Inputs=6
  Subsystem1 : Subsystem
  Subsystem2 : Subsystem
  Subsystem3 : Subsystem
  Subsystem4 : Subsystem
  Subsystem5 : Subsystem
  Subsystem6 : Subsystem
  u1 : PMIOPort  Side=Right
  u2 : PMIOPort  Port=2  Side=Right
  u3 : PMIOPort  Port=3  Side=Right
  u4 : PMIOPort  Port=4  Side=Right
  u5 : PMIOPort  Port=5  Side=Right
  u6 : PMIOPort  Port=6  Side=Right
  + : PMIOPort  Port=7  Side=Left
  - : PMIOPort  Port=8  Side=Left
  C : PMIOPort  Port=9  Side=Right
  torque : Outport  Unit=N*m
  motVel : Outport  Port=2  Unit=deg/s
  wires:
  [u6_tRef] -> Subsystem6/1(torqueCommand)  "u6_tRef"
  [u3_tRef] -> Subsystem3/1(torqueCommand)  "u3_tRef"
  Gain1/1 -> Mux1/2  "servo2w"
  [servo2_w] -> Gain1/1
  [servo6_w] -> Gain17/1
  [u2_tRef] -> Subsystem2/1(torqueCommand)  "u2_tRef"
  [servo1_w] -> Gain/1
  [servo4_w] -> Gain11/1
  Subsystem5/1(torque1) -> [servo5_t]  "torque"
  Subsystem4/2(motVel1) -> [servo4_w]  "motVel"
  Gain11/1 -> Mux1/4  "servo4w"
  Subsystem3/1(torque1) -> [servo3_t]  "torque"
  [servo3_w] -> Gain8/1
  [servo5_w] -> Gain14/1
  Subsystem6/2(motVel1) -> [servo6_w]  "motVel"
  Subsystem6/1(torque1) -> [servo6_t]  "torque"
  Subsystem3/2(motVel1) -> [servo3_w]  "motVel"
  Subsystem5/2(motVel1) -> [servo5_w]  "motVel"
  Gain/1 -> Mux1/1  "servo1w"
  Subsystem4/1(torque1) -> [servo4_t]  "torque"
  [u1_tRef] -> Subsystem1/1(torqueCommand)  "u1_tRef"
  Gain17/1 -> Mux1/6  "servo6w"
  Mux1/1 -> motVel/1
  Subsystem2/2(motVel1) -> [servo2_w]  "motVel"
  Subsystem2/1(torque1) -> [servo2_t]  "torque"
  Gain8/1 -> Mux1/3  "servo3w"
  [u5_tRef] -> Subsystem5/1(torqueCommand)  "u5_tRef"
  Subsystem1/1(torque1) -> [servo1_t]  "torque"
  [u4_tRef] -> Subsystem4/1(torqueCommand)  "u4_tRef"
  Subsystem1/2(motVel1) -> [servo1_w]  "motVel"
  Gain14/1 -> Mux1/5  "servo5w"
  Demux/1 -> [u1_tRef]
  Demux/2 -> [u2_tRef]
  Demux/3 -> [u3_tRef]
  Demux/4 -> [u4_tRef]
  Demux/5 -> [u5_tRef]
  Demux/6 -> [u6_tRef]
  tRef/1 -> Demux/1
  Mux/1 -> torque/1
  [servo1_t] -> Mux/1  "servo1t"
  [servo2_t] -> Mux/2  "servo2t"
  [servo3_t] -> Mux/3  "servo3t"
  [servo4_t] -> Mux/4  "servo4t"
  [servo5_t] -> Mux/5  "servo5t"
  [servo6_t] -> Mux/6  "servo6t"
  connections:
  Mechanical Rotational Reference5/LConn1 -- Subsystem6/RConn2
  u4/RConn1 -- Subsystem4/RConn1
  u3/RConn1 -- Subsystem3/RConn1
  u6/RConn1 -- Subsystem6/RConn1
  Subsystem1/LConn2 -- -/RConn1 -- Subsystem4/LConn2 -- Subsystem6/LConn2 -- Subsystem3/LConn2 -- Subsystem5/LConn2 -- Subsystem2/LConn2
  Mechanical Rotational Reference2/LConn1 -- Subsystem3/RConn2
  u2/RConn1 -- Subsystem2/RConn1
  Subsystem1/LConn1 -- +/RConn1 -- Subsystem5/LConn1 -- Subsystem3/LConn1 -- Subsystem6/LConn1 -- Subsystem2/LConn1 -- Subsystem4/LConn1
  u1/RConn1 -- Subsystem1/RConn1
  Mechanical Rotational Reference/LConn1 -- Subsystem1/RConn2
  Mechanical Rotational Reference1/LConn1 -- Subsystem2/RConn2
  Mechanical Rotational Reference4/LConn1 -- Subsystem5/RConn2
  u5/RConn1 -- Subsystem5/RConn1
  Subsystem4/RConn2 -- C/RConn1

== system IRB140_speed/Servomotor Position Controller/filter ==
  reference : Inport
  output : Inport  Port=2
  Low-Pass Filter (Discrete or Continuous) : eeGeneralControl/Low-Pass Filter (Discrete or Continuous)  K=1  T=0.01  B=inf  A=-inf  Ts=ts
      settings: SourceProductName=Simscape Electrical
  Sum : Sum  Inputs=|+-
  control : Outport
  wires:
  reference/1 -> Low-Pass Filter (Discrete or Continuous)/1
  output/1 -> Sum/2
  Low-Pass Filter (Discrete or Continuous)/1 -> Sum/1
  Sum/1 -> control/1

== system IRB140_speed/Servomotor Position Controller/filter1 ==
  reference : Inport
  output : Inport  Port=2
  Low-Pass Filter (Discrete or Continuous) : eeGeneralControl/Low-Pass Filter (Discrete or Continuous)  K=1  T=0.01  B=inf  A=-inf  Ts=ts
      settings: SourceProductName=Simscape Electrical
  Sum : Sum  Inputs=|+-
  control : Outport
  wires:
  reference/1 -> Low-Pass Filter (Discrete or Continuous)/1
  output/1 -> Sum/2
  Low-Pass Filter (Discrete or Continuous)/1 -> Sum/1
  Sum/1 -> control/1

== system IRB140_speed/Servomotor Position Controller/filter2 ==
  reference : Inport
  output : Inport  Port=2
  Low-Pass Filter (Discrete or Continuous) : eeGeneralControl/Low-Pass Filter (Discrete or Continuous)  K=1  T=0.01  B=inf  A=-inf  Ts=ts
      settings: SourceProductName=Simscape Electrical
  Sum : Sum  Inputs=|+-
  control : Outport
  wires:
  reference/1 -> Low-Pass Filter (Discrete or Continuous)/1
  output/1 -> Sum/2
  Low-Pass Filter (Discrete or Continuous)/1 -> Sum/1
  Sum/1 -> control/1

== system IRB140_speed/Servomotor Position Controller/filter3 ==
  reference : Inport
  output : Inport  Port=2
  Low-Pass Filter (Discrete or Continuous) : eeGeneralControl/Low-Pass Filter (Discrete or Continuous)  K=1  T=0.01  B=inf  A=-inf  Ts=ts
      settings: SourceProductName=Simscape Electrical
  Sum : Sum  Inputs=|+-
  control : Outport
  wires:
  reference/1 -> Low-Pass Filter (Discrete or Continuous)/1
  output/1 -> Sum/2
  Low-Pass Filter (Discrete or Continuous)/1 -> Sum/1
  Sum/1 -> control/1

== system IRB140_speed/Servomotor Position Controller/filter4 ==
  reference : Inport
  output : Inport  Port=2
  Low-Pass Filter (Discrete or Continuous) : eeGeneralControl/Low-Pass Filter (Discrete or Continuous)  K=1  T=0.01  B=inf  A=-inf  Ts=ts
      settings: SourceProductName=Simscape Electrical
  Sum : Sum  Inputs=|+-
  control : Outport
  wires:
  reference/1 -> Low-Pass Filter (Discrete or Continuous)/1
  output/1 -> Sum/2
  Low-Pass Filter (Discrete or Continuous)/1 -> Sum/1
  Sum/1 -> control/1

== system IRB140_speed/Servomotor Position Controller/filter5 ==
  reference : Inport
  output : Inport  Port=2
  Low-Pass Filter (Discrete or Continuous) : eeGeneralControl/Low-Pass Filter (Discrete or Continuous)  K=1  T=0.01  B=inf  A=-inf  Ts=ts
      settings: SourceProductName=Simscape Electrical
  Sum : Sum  Inputs=|+-
  control : Outport
  wires:
  reference/1 -> Low-Pass Filter (Discrete or Continuous)/1
  output/1 -> Sum/2
  Low-Pass Filter (Discrete or Continuous)/1 -> Sum/1
  Sum/1 -> control/1

== system IRB140_speed/Servomotor Speed Controller/filter ==
  reference : Inport
  output : Inport  Port=2
  Low-Pass Filter (Discrete or Continuous) : eeGeneralControl/Low-Pass Filter (Discrete or Continuous)  K=1  T=0.01  B=inf  A=-inf  Ts=ts
      settings: SourceProductName=Simscape Electrical
  Sum : Sum  Inputs=|+-
  control : Outport
  wires:
  reference/1 -> Low-Pass Filter (Discrete or Continuous)/1
  output/1 -> Sum/2
  Low-Pass Filter (Discrete or Continuous)/1 -> Sum/1
  Sum/1 -> control/1

== system IRB140_speed/Servomotor Speed Controller/filter1 ==
  reference : Inport
  output : Inport  Port=2
  Low-Pass Filter (Discrete or Continuous) : eeGeneralControl/Low-Pass Filter (Discrete or Continuous)  K=1  T=0.01  B=inf  A=-inf  Ts=ts
      settings: SourceProductName=Simscape Electrical
  Sum : Sum  Inputs=|+-
  control : Outport
  wires:
  reference/1 -> Low-Pass Filter (Discrete or Continuous)/1
  output/1 -> Sum/2
  Low-Pass Filter (Discrete or Continuous)/1 -> Sum/1
  Sum/1 -> control/1

== system IRB140_speed/Servomotor Speed Controller/filter2 ==
  reference : Inport
  output : Inport  Port=2
  Low-Pass Filter (Discrete or Continuous) : eeGeneralControl/Low-Pass Filter (Discrete or Continuous)  K=1  T=0.01  B=inf  A=-inf  Ts=ts
      settings: SourceProductName=Simscape Electrical
  Sum : Sum  Inputs=|+-
  control : Outport
  wires:
  reference/1 -> Low-Pass Filter (Discrete or Continuous)/1
  output/1 -> Sum/2
  Low-Pass Filter (Discrete or Continuous)/1 -> Sum/1
  Sum/1 -> control/1

== system IRB140_speed/Servomotor Speed Controller/filter3 ==
  reference : Inport
  output : Inport  Port=2
  Low-Pass Filter (Discrete or Continuous) : eeGeneralControl/Low-Pass Filter (Discrete or Continuous)  K=1  T=0.01  B=inf  A=-inf  Ts=ts
      settings: SourceProductName=Simscape Electrical
  Sum : Sum  Inputs=|+-
  control : Outport
  wires:
  reference/1 -> Low-Pass Filter (Discrete or Continuous)/1
  output/1 -> Sum/2
  Low-Pass Filter (Discrete or Continuous)/1 -> Sum/1
  Sum/1 -> control/1

== system IRB140_speed/Servomotor Speed Controller/filter4 ==
  reference : Inport
  output : Inport  Port=2
  Low-Pass Filter (Discrete or Continuous) : eeGeneralControl/Low-Pass Filter (Discrete or Continuous)  K=1  T=0.01  B=inf  A=-inf  Ts=ts
      settings: SourceProductName=Simscape Electrical
  Sum : Sum  Inputs=|+-
  control : Outport
  wires:
  reference/1 -> Low-Pass Filter (Discrete or Continuous)/1
  output/1 -> Sum/2
  Low-Pass Filter (Discrete or Continuous)/1 -> Sum/1
  Sum/1 -> control/1

== system IRB140_speed/Servomotor Speed Controller/filter5 ==
  reference : Inport
  output : Inport  Port=2
  Low-Pass Filter (Discrete or Continuous) : eeGeneralControl/Low-Pass Filter (Discrete or Continuous)  K=1  T=0.01  B=inf  A=-inf  Ts=ts
      settings: SourceProductName=Simscape Electrical
  Sum : Sum  Inputs=|+-
  control : Outport
  wires:
  reference/1 -> Low-Pass Filter (Discrete or Continuous)/1
  output/1 -> Sum/2
  Low-Pass Filter (Discrete or Continuous)/1 -> Sum/1
  Sum/1 -> control/1

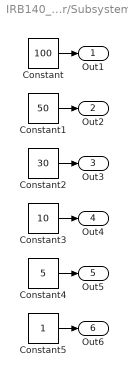
== system IRB140_speed/r/Subsystem ==
  Constant : Constant  Value=100
  Constant1 : Constant  Value=50
  Constant2 : Constant  Value=30
  Constant3 : Constant  Value=10
  Constant4 : Constant  Value=5
  Constant5 : Constant
  Out1 : Outport
  Out2 : Outport  Port=2
  Out3 : Outport  Port=3
  Out4 : Outport  Port=4
  Out5 : Outport  Port=5
  Out6 : Outport  Port=6
  wires:
  Constant3/1 -> Out4/1
  Constant1/1 -> Out2/1
  Constant4/1 -> Out5/1
  Constant5/1 -> Out6/1
  Constant2/1 -> Out3/1
  Constant/1 -> Out1/1

== system IRB140_speed/r/Trajectories1 ==
  Demux : Demux  Tag=STV Demux  Outputs=6
  FromWs : FromWorkspace  Tag=STV FromWs  VariableName=tuvar  SampleTime=0
      SigBuilderData=|
      | common.afterFinalStr = 'Extrapolate'
      | common.sampleTime = '0'
      | dataSet.timeRange = [0 20]
      | dataSet.name = 'jointMotion'
      | sbobj.Groups.Name = 'jointMotion'
      | sbobj.Groups.Signals(1).Name = 'servopos1'
      | sbobj.Groups.Signals(1).XData = [0 2.5 7.5 12.5 17.5 20]
      | sbobj.Groups.Signals(1).YData = [0 50 48 86 86 0]
      | sbobj.Groups.Signals(2).Name = 'servopos2'
      | sbobj.Groups.Signals(2).XData = [0 2.5 7.5 12.5 17.5 20]
      | sbobj.Groups.Signals(2).YData = [0 0 52 52 0 0]
      | sbobj.Groups.Signals(3).Name = 'servopos3'
      | sbobj.Groups.Signals(3).XData = [0 2.5 4.5 5.5 7.5 12.5 14.5 15.5 17.5 20]
      | sbobj.Groups.Signals(3).YData = [0 0 100 100 0 0 105 105 0 0]
      | sbobj.Groups.Signals(4).Name = 'servopos4'
      | sbobj.Groups.Signals(4).XData = [0 2.5 4.5 5.5 7.5 12.5 14.5 15.5 17.5 20]
      | sbobj.Groups.Signals(4).YData = [0 0 45 45 0 0 34 34 0 0]
      | sbobj.Groups.Signals(5).Name = 'servopos5'
      | sbobj.Groups.Signals(5).XData = [0 4 4.5 5.5 6 14.5 15.5 20]
      | sbobj.Groups.Signals(5).YData = [136 136 136 150 150 150 136 136]
      | sbobj.Groups.Signals(6).Name = 'servopos6'
      | sbobj.Groups.Signals(6).XData = [0 4 4.5 5.5 6 14.5 15.5 20]
      | sbobj.Groups.Signals(6).YData = [24 25 95 95 30 30 100 100]
      | sbobj.Groups.TimeRange = [0 20]
  servopos1 : Outport  Tag=STV Outport
  servopos2 : Outport  Tag=STV Outport  Port=2
  servopos3 : Outport  Tag=STV Outport  Port=3
  servopos4 : Outport  Tag=STV Outport  Port=4
  servopos5 : Outport  Tag=STV Outport  Port=5
  servopos6 : Outport  Tag=STV Outport  Port=6
  wires:
  FromWs/1 -> Demux/1
  Demux/1 -> servopos1/1
  Demux/2 -> servopos2/1
  Demux/3 -> servopos3/1
  Demux/4 -> servopos4/1
  Demux/5 -> servopos5/1
  Demux/6 -> servopos6/1

== system IRB140_speed/Plant/robot/Subsystem ==
  joint1 : sm_lib/Joints/Revolute Joint  SenseConstraintForce=off  SenseConstraintForceX=off  SenseConstraintForceY=off  SenseConstraintForceZ=off  SenseConstraintTorque=off  SenseConstraintTorqueX=off  SenseConstraintTorqueY=off  SenseConstraintTorqueZ=off  SenseTotalForce=off  SenseTotalForceX=off  SenseTotalForceY=off  SenseTotalForceZ=off  SenseTotalTorque=off  SenseTotalTorqueX=off  SenseTotalTorqueY=off  SenseTotalTorqueZ=off  CompositeWrenchDir=FollowerOnBase  CompositeWrenchFrame=BaseFrame  EquilibriumPosition=0  EquilibriumPositionUnits=deg  SpringStiffness=0  SpringStiffnessUnits=N*m/deg  DampingCoefficient=0  DampingCoefficientUnits=m^2*kg/s/rad  TorqueActuationMode=InputTorque  MotionActuationMode=ComputedMotion  SensePosition=on  SenseVelocity=on  SenseAcceleration=off  SenseTorqueForce=off  SenseLowerLimitTorqueForce=off  SenseUpperLimitTorqueForce=off  LowerLimitSpecify=off  LowerLimitBound=-90  LowerLimitBoundUnits=deg  LowerLimitStiffness=1e4  LowerLimitStiffnessUnits=N*m/deg  LowerLimitDamping=10  LowerLimitDampingUnits=N*m/(deg/s)  LowerLimitTransitionRegionWidth=0.1  LowerLimitTransitionRegionWidthUnits=deg  UpperLimitSpecify=off  UpperLimitBound=90  UpperLimitBoundUnits=deg  UpperLimitStiffness=1e4  UpperLimitStiffnessUnits=N*m/deg  UpperLimitDamping=10  UpperLimitDampingUnits=N*m/(deg/s)  UpperLimitTransitionRegionWidth=0.1  UpperLimitTransitionRegionWidthUnits=deg  PositionTargetSpecify=on  PositionTargetPriority=Low  PositionTargetValue=0  PositionTargetValueUnits=deg  VelocityTargetSpecify=off  VelocityTargetPriority=High  VelocityTargetValue=0  VelocityTargetValueUnits=deg/s
  "rot2rev " : Subsystem
  B : PMIOPort  Side=Left
  F : PMIOPort  Port=2  Side=Right
  q : PMIOPort  Port=3  Side=Right
  w : PMIOPort  Port=4  Side=Right
  C : PMIOPort  Port=5  Side=Left
  R : PMIOPort  Port=6  Side=Right
  connections:
  joint1/RConn2 -- q/RConn1
  joint1/RConn3 -- "rot2rev "/RConn1 -- w/RConn1
  joint1/LConn2 -- "rot2rev "/LConn1
  joint1/RConn1 -- F/RConn1
  B/RConn1 -- joint1/LConn1
  C/RConn1 -- "rot2rev "/LConn2
  "rot2rev "/RConn2 -- R/RConn1
